simulink model "main"  (R2016b)
settings: Solver=FixedStepAuto  StartTime=0.0  StopTime=10.0  RelTol=1e-3
libraries: embdlinuxlib x2, etargetslib x1
settings Model: Creator=abz  LastModifiedBy=abz
settings SolverCC: PositivePriorityOrder=on
settings OptimizationCC: MaxStackSize=64
settings DebuggingCC: ParameterTunabilityLossMsg=error
settings HardwareCC: ProdBitPerPointer=32  ProdBitPerSizeT=32  ProdBitPerPtrDiffT=32  ProdLargestAtomicInteger=Long  ProdLargestAtomicFloat=Double  ProdWordSize=32  ProdHWDeviceType=ARM Compatible->ARM Cortex
settings RTWCC: SystemTargetFile=ert.tlc  HardwareBoard=Raspberry Pi  TLCOptions="-aInlineSetEventsForThisBaseRateFcn=TLC_FALSE -aSuppressMultiTaskScheduler=TLC_FALSE  -aRateBasedStepFcn=0"  TemplateMakefile=ert_default_tmf  Description=Embedded Coder  GenerateReport=on  Toolchain=GNU GCC Raspberry Pi  IncludeHyperlinkInReport=on  LaunchReport=on  GenerateTraceInfo=on  GenerateTraceReport=on  GenerateTraceReportSl=on  GenerateTraceReportSf=on  GenerateTraceReportEml=on
settings CodeAppCC: ForceParamTrailComments=on  IgnoreCustomStorageClasses=off  OperatorAnnotations=on  SimulinkDataObjDesc=on  SFDataObjDesc=on  MATLABFcnDesc=on  InsertBlockDesc=on  MATLABSourceComments=on
settings ERTTargetCC: SupportVariableSizeSignals=on

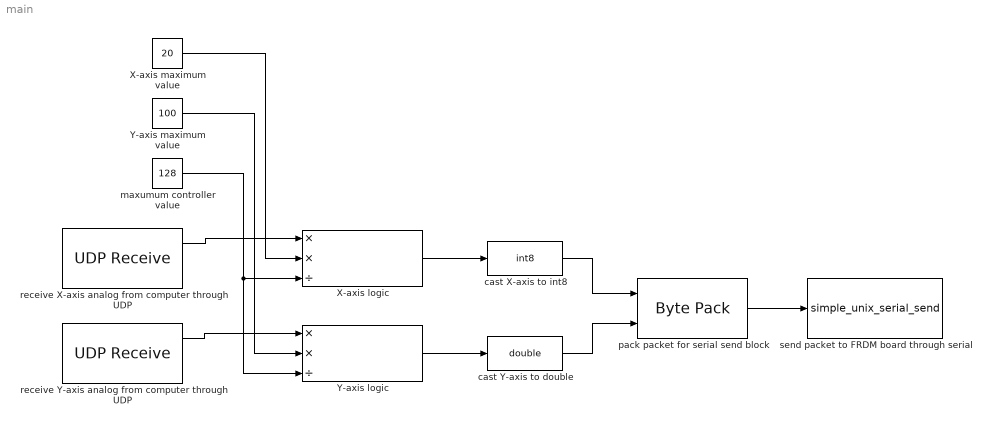
== system main ==
  X-axis logic : Product  Inputs=**/
  X-axis maximum value : Constant  Value=20
  Y-axis logic : Product  Inputs=**/
  Y-axis maximum value : Constant  Value=100
  cast X-axis to int8 : DataTypeConversion  OutDataTypeStr=int8
  cast Y-axis to double : DataTypeConversion  OutDataTypeStr=double
  maxumum controller value : Constant  Value=128
  pack packet for serial send block : etargetslib/Byte Pack  datatypes={'int8', 'double'}  byteAlign=1
  receive X-axis analog from computer through UDP : embdlinuxlib/UDP Receive  localURL='0.0.0.0'  localPort=20001  remoteURL='0.0.0.0'  remotePort=-1  recvBufferSize=8192  signalDatatype=int8  dims=1  isVarSize=off  showBlockingTime=off  blockingTime=0  sampletime=0.01  blockPlatform=Raspberry Pi
  receive Y-axis analog from computer through UDP : embdlinuxlib/UDP Receive  localURL='0.0.0.0'  localPort=20000  remoteURL='0.0.0.0'  remotePort=-1  recvBufferSize=8192  signalDatatype=int8  dims=1  isVarSize=off  showBlockingTime=off  blockingTime=0  sampletime=0.01  blockPlatform=Raspberry Pi
  send packet to FRDM board through serial : S-Function  FunctionName=simple_unix_serial_send  SFunctionModules='simple_unix_serial_send'  SFunctionDeploymentMode=off  EnableBusSupport=off
  wires:
  receive X-axis analog from computer through UDP/1 -> X-axis logic/1
  maxumum controller value/1 -> X-axis logic/3, Y-axis logic/3
  receive Y-axis analog from computer through UDP/1 -> Y-axis logic/1
  X-axis maximum value/1 -> X-axis logic/2
  Y-axis maximum value/1 -> Y-axis logic/2
  pack packet for serial send block/1 -> send packet to FRDM board through serial/1
  Y-axis logic/1 -> cast Y-axis to double/1
  cast Y-axis to double/1 -> pack packet for serial send block/2
  cast X-axis to int8/1 -> pack packet for serial send block/1
  X-axis logic/1 -> cast X-axis to int8/1
